simulink model "highGturnSim"  (R2023b)
settings: Solver=VariableStepAuto  StartTime=0.0  StopTime=10  FixedStep=0.01  RelTol=1e-3
libraries: aerolibconvert2 x1, aerolibactuator x1
settings Model: Creator=vanha  LastModifiedBy=vanha

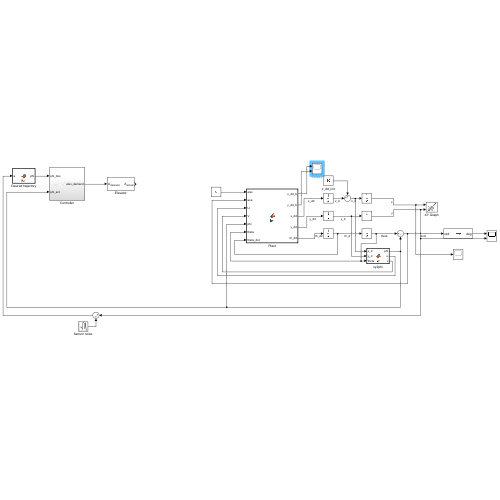
[thumbnail: Simulink's stored preview of the top-level diagram]
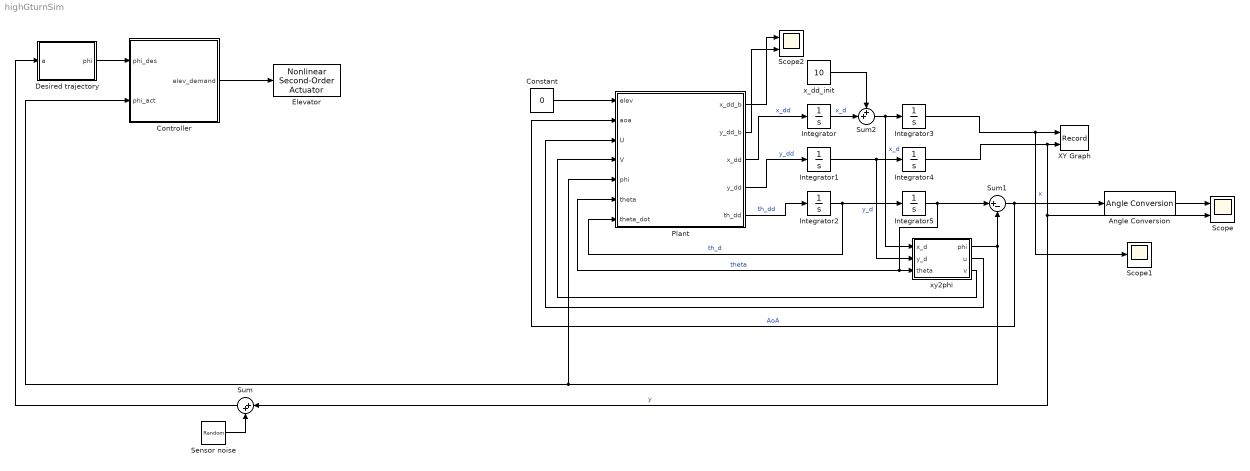
== system highGturnSim ==
  Angle Conversion : aerolibconvert2/Angle Conversion  IU=rad  OU=deg
  Constant : Constant  Value=0
  Controller : Subsystem
  Desired trajectory : MATLAB Function  TreatAsAtomicUnit=on
  Elevator : aerolibactuator/Nonlinear Second-Order Actuator  wn_fin=1  z_fin=0.3  fin_max=deg2rad(10)  fin_min=-deg2rad(30)  fin_maxrate=500*pi/180  fin_act_0=0  fin_act_vel=0
  Integrator{,1..5} (6 alike) : Integrator
  Plant : MATLAB Function  TreatAsAtomicUnit=on
  Scope : Scope  NumInputPorts=2
  Scope1 : Scope
  Scope2 : Scope  NumInputPorts=2
  Sensor noise : RandomNumber  Variance=0.25  SampleTime=0.1
  Sum : Sum  Inputs=|++
  Sum1 : Sum  Inputs=|+-
  Sum2 : Sum  Inputs=++|
  XY Graph : Record  FileSettingsInternal="{\"entries\":[{\"content\":{\"excelSettings\":{\"content\":{},\"type\":\"Streamout.ExcelSettings\"}},\"type\":\"Streamout.FileSettingStorage\",\"uuid\":\"\"}],\"packageUris\":[\"http:\\/\\/schema.mathworks.com\\/mf0\\/streamout_blocks\\/R2020a\"],\"version\":\"1.0\"}"  Layout=[1 1]  SignalsInternal="{\"entries\":[{\"content\":{\"signals\":[{\"content\":{\"blockPath\":[],\"dimensions\":[1],\"domain\":\"\",\"lineColor\":\"#a2142f\",\"plots\":[1],\"port\":1,\"sid\":[\"\"],\"signalID\":391,\"signalName\":\"x\"},\"type\":\"RecordBlkView.Signal\",\"uuid\":\"\"},{\"content\":{\"blockPath\":[],\"dimensions\":[1],\"domain\":\"\",\"lineColor\":\"#139fff\",\"plots\":[1],\"port\":2,\"sid\":[\"\"],\"signalID\":395,\"signalName\":\"y\"},\"type\":\"RecordBlkView.Signal\",\"uuid\":\"\"}]},\"type\":\"RecordBlkView.InputSignals\",\"uuid\":\"\"}],\"packageUris\":[\"http:\\/\\/schema.mathworks.com\\/mf0\\/streamout_blocks\\/R2020a\"],\"version\":\"1.0\"}"  VisualizationBindings="{\"xyplotplugin\":{\"info\":[{\"series\":[{\"bindingParametersList\":[{\"parameter\":\"X-Axis\",\"signalID\":391,\"signalName\":\"x\"},{\"parameter\":\"Y-Axis\",\"signalID\":395,\"signalName\":\"y\"}],\"seriesID\":51392}],\"subplotID\":1}]}}"  CompatibilityTag=XY
  x_dd_init : Constant  Value=10
  xy2phi : MATLAB Function  TreatAsAtomicUnit=on
  wires:
  Sensor noise/1 -> Sum/2
  Sum/1 -> Desired trajectory/1(a)
  Controller/1(elev_demand) -> Elevator/1
  Plant/3(x_dd) -> Integrator/1  "x_dd"
  Plant/4(y_dd) -> Integrator1/1  "y_dd"
  Plant/5(th_dd) -> Integrator2/1  "th_dd"
  Sum2/1 -> xy2phi/1(x_d), Integrator3/1  "x_d"
  Integrator1/1 -> xy2phi/2(y_d), Integrator4/1  "y_d"
  Integrator2/1 -> Plant/7(theta_dot), Integrator5/1  "th_d"
  Integrator3/1 -> Scope1/1, XY Graph/1  "x"
  Integrator4/1 -> Scope/2, Sum/1, XY Graph/2  "y"
  Integrator5/1 -> Plant/6(theta), xy2phi/3(theta), Sum1/1  "theta"
  Desired trajectory/1(phi) -> Controller/1(phi_des)
  xy2phi/1(phi) -> Plant/5(phi), Controller/2(phi_act), Sum1/2
  Sum1/1 -> Angle Conversion/1, Plant/2(aoa)  "AoA"
  xy2phi/2(u) -> Plant/3(U)
  xy2phi/3(v) -> Plant/4(V)
  Constant/1 -> Plant/1(elev)
  Integrator/1 -> Sum2/2  "x_d"
  x_dd_init/1 -> Sum2/1
  Angle Conversion/1 -> Scope/1
  Plant/1(x_dd_b) -> Scope2/1
  Plant/2(y_dd_b) -> Scope2/2

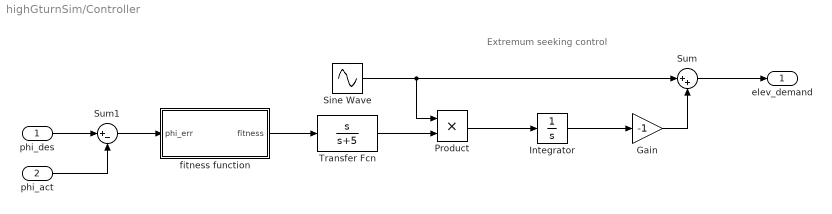
== system highGturnSim/Controller ==
  note: Extremum seeking control
  phi_des : Inport
  phi_act : Inport  Port=2
  Gain : Gain  Gain=-1
  Integrator : Integrator
  Product : Product
  Sine Wave : Sin  SampleTime=0
  Sum : Sum  Inputs=|++
  Sum1 : Sum  Inputs=|+-
  Transfer Fcn : TransferFcn  Numerator=[1 0]  Denominator=[1 5]
  fitness function : MATLAB Function  TreatAsAtomicUnit=on
  elev_demand : Outport
  wires:
  Sine Wave/1 -> Sum/1, Product/1
  Product/1 -> Integrator/1
  Integrator/1 -> Gain/1
  Gain/1 -> Sum/2
  phi_des/1 -> Sum1/1
  phi_act/1 -> Sum1/2
  Sum1/1 -> fitness function/1(phi_err)
  fitness function/1(fitness) -> Transfer Fcn/1
  Transfer Fcn/1 -> Product/2
  Sum/1 -> elev_demand/1

== matlab function highGturnSim/Plant ==
  data: x_dd_b output; y_dd_b output; elev input; x_dd output; y_dd output; th_dd output; aoa input; U input; V input; phi input; theta input; theta_dot input
function [x_dd_b,y_dd_b,x_dd,y_dd,th_dd] = fcn(elev,aoa,U,V,phi,theta,theta_dot)

b = 1; %wingspan (m)
b_tail = 0.3; %tailspan
AR = 5; %aspect ratio
AR_tail = 3; %tail aspect ratio
I = 1; %moment of inertia (kg-m^2)
rho = 1.225; %air density (kg/m^3)
oswald = 0.9; %Oswald efficiency ratio
camber_number = 2; %NACA 4 digit airfoil camber amount number (used for lift coefficient approximation)
VH = 1;
m = 2; %mass (kg)

% flight coefficients and derivatives
dCLtdelev = 0.04; %Change in lift of tail wrt to change in elevator angle
dcmdaoa = -0.0133; %change in moment wrt to aoa
C_M0 = 0.06; %profile moment

c_mn = b/AR; %mean chord length (m)
S_main = c_mn*b; %Planform area (m^2)

c_mn_tail = b_tail/AR_tail; %mean chord length of tail (m)
S_tail = c_mn_tail*b_tail; %planform area of tail (m^2)

%% Coefficients of flight
a0 = 2*pi; %infinite wing lift slope approximation (1/rad)
C_l0 = a0*deg2rad(camber_number); %profile lift coefficient
a = a0/(1+a0/(pi*oswald*AR)); %finite wing lift slope approximation (1/rad)
C_L = a*aoa+C_l0; %Finite wing lift coefficient
a_tail = a0/(1+a0/(pi*oswald*AR_tail));
C_Ltail = a_tail*aoa+dCLtdelev*elev;

C_d_profile = 0.02; %profile drag coefficient
C_D = C_d_profile + (C_L*C_L)/(pi*oswald*AR); %Finite wing drag coefficient

C_M = C_M0+dcmdaoa*aoa-VH*dCLtdelev*elev; %Moment coefficient

%% Calculate lift/drag/moment
V_mag = sqrt(U^2+V^2); %velocity magnitude (m/s)
q = rho*V_mag*V_mag/2; %dynamic pressure (pa)

L = q*(C_L*S_main+C_Ltail*S_tail); %Lift (N)
D = q*C_D*S_main; %Drag (N)
M = q*C_M*S_main*c_mn; %Moment (N-m)

%% Equations of motion
G = [cos(theta),-sin(theta);sin(theta),cos(theta)]*[0;-9.81*m];

Udot = G(1)-D;
Vdot = G(2)+L;

x_dd_b = Udot+theta_dot*V;
y_dd_b = Vdot;

%motion in global frame
x_dd = x_dd_b*cos(theta)+y_dd_b*sin(theta);
y_dd = y_dd_b*cos(theta)+x_dd_b*sin(theta);
th_dd = M/I;

end

== matlab function highGturnSim/xy2phi ==
  data: x_d input; phi output; y_d input; theta input; u output; v output
function [phi,u,v] = fcn(x_d,y_d,theta)

phi = atan2(y_d,x_d);
u = x_d*cos(theta)+y_d*sin(theta);
v = y_d*cos(theta)-x_d*sin(theta);

== matlab function highGturnSim/Desired trajectory ==
  data: phi output; a input
function phi = fcn(a) %a is altitude, theta is velocity angle

%r = 100; %turn radius in meters

phi = 0;

== matlab function highGturnSim/Controller/fitness function ==
  data: phi_err input; fitness output
function fitness = fcn(phi_err)

%we want to minimize the fitness function
A = 1;
fitness = A*phi_err^2;
